simulink model "PID_control_heat_pump"  (R2016a)
settings: Solver=VariableStepAuto  StartTime=0.0  StopTime=50  RelTol=1e-3
libraries: fuzblock x1, simulink x1
settings Model: Creator=EBUKA  LastModifiedBy=EBUKA

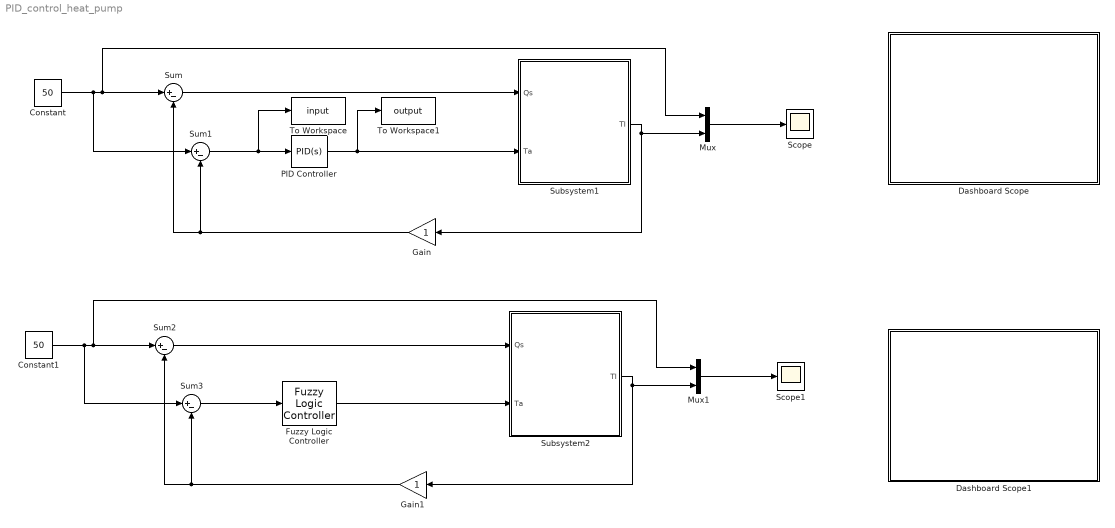
== system PID_control_heat_pump ==
  Constant : Constant  Value=50
  Constant1 : Constant  Value=50
  Dashboard Scope : Subsystem  DialogController=hmiCreateDDGDialog  IsWebBlock=on  mask(MWDashboardBlock){webBlockId=cb9a7734-cccb-488b-b28e-750a8465cbea, webBlockType=sdiscope, ShowInitialText=on, HMISrcModelName=PID_control_heat_pump}
      mask prompts: webBlockId "WebBlock Id"; webBlockType "WebBlock Type"; HMISrcModelName "Source Model"
      mask Help: helpview([docroot '/mapfiles/simulink.map'], 'hmi_scope')
      mask Display:
      | if strcmp(get_param(bdroot(gcb),'BlockDiagramType'), 'library')
      |     image([(matlabroot) '/toolbox/simulink/hmi/icons/DashboardScope.png']);
      | end
  Dashboard Scope1 : Subsystem  DialogController=hmiCreateDDGDialog  IsWebBlock=on  mask(MWDashboardBlock){webBlockId=57892931-2b63-466b-bcf0-821fd85189da, webBlockType=sdiscope, ShowInitialText=on, HMISrcModelName=PID_control_heat_pump}
      mask prompts: webBlockId "WebBlock Id"; webBlockType "WebBlock Type"; HMISrcModelName "Source Model"
      mask Help: helpview([docroot '/mapfiles/simulink.map'], 'hmi_scope')
      mask Display:
      | if strcmp(get_param(bdroot(gcb),'BlockDiagramType'), 'library')
      |     image([(matlabroot) '/toolbox/simulink/hmi/icons/DashboardScope.png']);
      | end
  Fuzzy Logic Controller : fuzblock/Fuzzy Logic  Controller  fis=Temp
  Gain : Gain
  Gain1 : Gain
  Mux : Mux  Inputs=2
  Mux1 : Mux  Inputs=2
  PID Controller : simulink/Continuous/PID Controller  Controller=PID  TimeDomain=Continuous-time  SampleTime=-1  IntegratorMethod=Forward Euler  FilterMethod=Forward Euler  Form=Parallel  UseFilter=on  ControllerParametersSource=internal  P=1.575  I=2.5  D=0  N=100  InitialConditionSource=internal  InitialConditionForIntegrator=0  InitialConditionForFilter=0  ExternalReset=none  LimitOutput=off  UpperSaturationLimit=inf  LowerSaturationLimit=-inf  LinearizeAsGain=on  AntiWindupMode=none  Kb=1  TrackingMode=off  Kt=1  PParamMin=[]  PParamMax=[]  IParamMin=[]  IParamMax=[]  DParamMin=[]  DParamMax=[]  NParamMin=[]  NParamMax=[]  KbParamMin=[]  KbParamMax=[]  KtParamMin=[]  KtParamMax=[]  POutMin=[]  POutMax=[]  IOutMin=[]  IOutMax=[]  DOutMin=[]  DOutMax=[]  NOutMin=[]  NOutMax=[]  KbOutMin=[]  KbOutMax=[]  KtOutMin=[]  KtOutMax=[]  IntegratorOutMin=[]  IntegratorOutMax=[]  FilterOutMin=[]  FilterOutMax=[]  SumOutMin=[]  SumOutMax=[]  SumI1OutMin=[]  SumI1OutMax=[]  SumI2OutMin=[]  SumI2OutMax=[]  SumI3OutMin=[]  SumI3OutMax=[]  SumDOutMin=[]  SumDOutMax=[]  SaturationOutMin=[]  SaturationOutMax=[]  IntegratorContinuousStateAttributes=''  IntegratorStateMustResolveToSignalObject=off  IntegratorRTWStateStorageClass=Auto  FilterContinuousStateAttributes=''  FilterStateMustResolveToSignalObject=off  FilterRTWStateStorageClass=Auto  DifferentiatorICPrevScaledInput=0  DifferentiatorOutMin=[]  DifferentiatorOutMax=[]
  Scope : Scope
  Scope1 : Scope
  Subsystem1 : Subsystem
  Subsystem2 : Subsystem
  Sum{,1..3} (4 alike) : Sum  Inputs=|+-
  To Workspace : ToWorkspace  VariableName=input  SaveFormat=Timeseries  SampleTime=-1
  To Workspace1 : ToWorkspace  VariableName=output  SaveFormat=Timeseries  SampleTime=-1
  wires:
  Constant/1 -> Sum1/1, Mux/1, Sum/1
  Subsystem1/1(TI) -> Mux/2, Gain/1
  Sum/1 -> Subsystem1/1(Qs)
  PID Controller/1 -> To Workspace1/1, Subsystem1/2(Ta)
  Gain/1 -> Sum1/2, Sum/2
  Sum1/1 -> To Workspace/1, PID Controller/1
  Mux/1 -> Scope/1
  Constant1/1 -> Sum3/1, Mux1/1, Sum2/1
  Subsystem2/1(TI) -> Mux1/2, Gain1/1
  Sum2/1 -> Subsystem2/1(Qs)
  Fuzzy Logic Controller/1 -> Subsystem2/2(Ta)
  Gain1/1 -> Sum3/2, Sum2/2
  Sum3/1 -> Fuzzy Logic Controller/1
  Mux1/1 -> Scope1/1

== system PID_control_heat_pump/Dashboard Scope ==

== system PID_control_heat_pump/Dashboard Scope1 ==

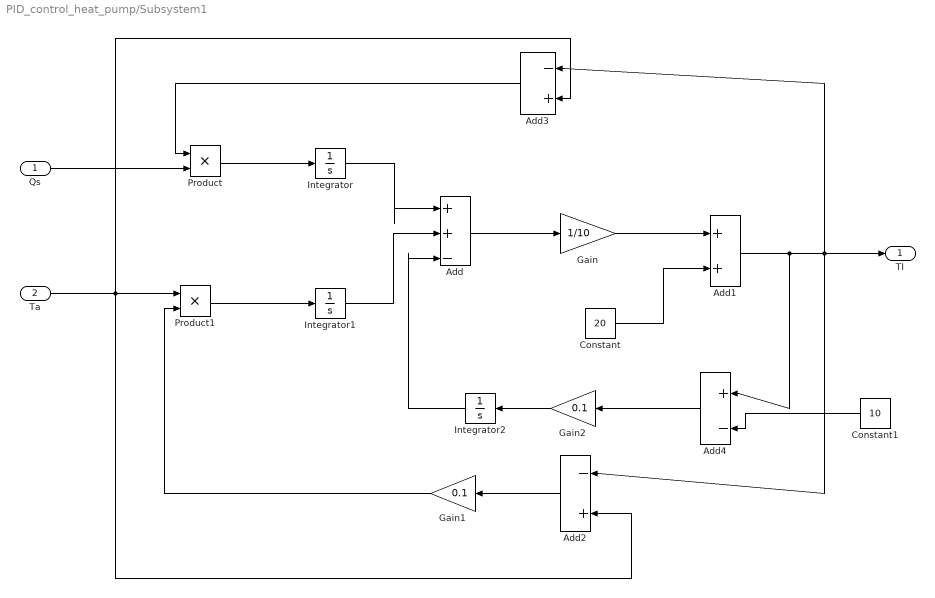
== system PID_control_heat_pump/Subsystem1 ==
  Qs : Inport
  Ta : Inport  Port=2
  Add : Sum  Inputs=|++-
  Add1 : Sum
  Add2 : Sum  Inputs=|-+
  Add3 : Sum  Inputs=|-+
  Add4 : Sum  Inputs=|+-
  Constant : Constant  Value=20
  Constant1 : Constant  Value=10
  Gain : Gain  Gain=1/10
  Gain1 : Gain  Gain=0.1
  Gain2 : Gain  Gain=0.1
  Integrator : Integrator
  Integrator1 : Integrator
  Integrator2 : Integrator
  Product : Product
  Product1 : Product
  TI : Outport
  wires:
  Add2/1 -> Gain1/1
  Gain1/1 -> Product1/2
  Qs/1 -> Product/2
  Integrator1/1 -> Add/2
  Product/1 -> Integrator/1
  Add/1 -> Gain/1
  Constant1/1 -> Add4/2
  Add4/1 -> Gain2/1
  Gain/1 -> Add1/1
  Gain2/1 -> Integrator2/1
  Integrator2/1 -> Add/3
  Ta/1 -> Add3/2, Add2/2, Product1/1
  Constant/1 -> Add1/2
  Add1/1 -> Add4/1, TI/1, Add3/1, Add2/1
  Integrator/1 -> Add/1
  Product1/1 -> Integrator1/1
  Add3/1 -> Product/1

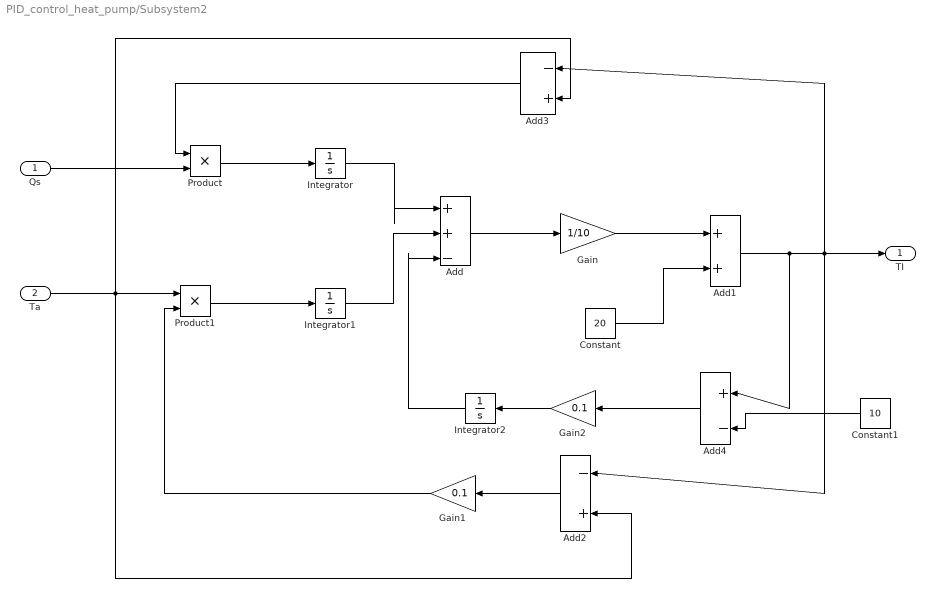
== system PID_control_heat_pump/Subsystem2 ==
  Qs : Inport
  Ta : Inport  Port=2
  Add : Sum  Inputs=|++-
  Add1 : Sum
  Add2 : Sum  Inputs=|-+
  Add3 : Sum  Inputs=|-+
  Add4 : Sum  Inputs=|+-
  Constant : Constant  Value=20
  Constant1 : Constant  Value=10
  Gain : Gain  Gain=1/10
  Gain1 : Gain  Gain=0.1
  Gain2 : Gain  Gain=0.1
  Integrator : Integrator
  Integrator1 : Integrator
  Integrator2 : Integrator
  Product : Product
  Product1 : Product
  TI : Outport
  wires:
  Add2/1 -> Gain1/1
  Gain1/1 -> Product1/2
  Qs/1 -> Product/2
  Integrator1/1 -> Add/2
  Product/1 -> Integrator/1
  Add/1 -> Gain/1
  Constant1/1 -> Add4/2
  Add4/1 -> Gain2/1
  Gain/1 -> Add1/1
  Gain2/1 -> Integrator2/1
  Integrator2/1 -> Add/3
  Ta/1 -> Add3/2, Add2/2, Product1/1
  Constant/1 -> Add1/2
  Add1/1 -> Add4/1, TI/1, Add3/1, Add2/1
  Integrator/1 -> Add/1
  Product1/1 -> Integrator1/1
  Add3/1 -> Product/1
